simulink model "a6_"  (R2012b)
settings: Solver=ode45  StartTime=0.0  StopTime=40.0  MaxStep=0.01  RelTol=1e-3
values from neighbouring files (symbols this model uses):
  K0 = 10^(11.4/20)    (= 3.71535229097)    [a6_.m]
settings Model: Creator=andre.bergmann  LastModifiedBy=andre.bergmann

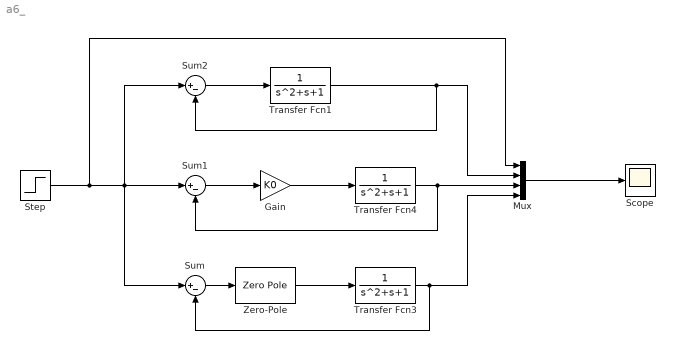
== system a6_ ==
  Gain : Gain  Gain=K0
  Mux : Mux
  Scope : Scope
  Step : Step  SampleTime=0
  Sum : Sum  Inputs=|+-
  Sum1 : Sum  Inputs=|+-
  Sum2 : Sum  Inputs=|+-
  Transfer Fcn1 : TransferFcn  Denominator=[1 1 1]
  Transfer Fcn3 : TransferFcn  Denominator=[1 1 1]
  Transfer Fcn4 : TransferFcn  Denominator=[1 1 1]
  Zero-Pole : ZeroPole  Zeros=[-0.15]  Poles=[-0.003]  Gain=[1.95]
  wires:
  Step/1 -> Mux/1, Sum/1, Sum2/1, Sum1/1
  Sum2/1 -> Transfer Fcn1/1
  Transfer Fcn1/1 -> Sum2/2, Mux/2
  Sum1/1 -> Gain/1
  Gain/1 -> Transfer Fcn4/1
  Transfer Fcn4/1 -> Sum1/2, Mux/3
  Transfer Fcn3/1 -> Mux/4, Sum/2
  Zero-Pole/1 -> Transfer Fcn3/1
  Sum/1 -> Zero-Pole/1
  Mux/1 -> Scope/1
